simulink model "CorrectionAlgorithmHorizontalAndVertical"  (R2023a)
settings: Solver=FixedStepDiscrete  StartTime=0.0  StopTime=2  RelTol=1e-3
undefined symbols (not defined in the file or in its folder): gray
libraries: simulink x20, hdlsllib x10, visionsources x8, visionhdlio x6, dspsigops x4, visionhdlutilities x1
Description:
  | Sobel Edge Detection Using the MATLAB(R) Function Block
  | This example shows how to use HDL Coder(TM) to check,
  | generate, and verify HDL code for a Sobel Edge Detection
  | block built using the MATLAB Function block.
settings Model: Creator=The MathWorks, Inc.  LastModifiedBy=jms7664
settings SolverCC: AlgebraicLoopSolver=TrustRegion
settings DataIOCC: LimitDataPoints=on  SaveFormat=Array  SignalLogging=off  ReturnWorkspaceOutputs=off
settings OptimizationCC: BlockReduction=off  ConditionallyExecuteInputs=off  DefaultParameterBehavior=Inlined  ExpressionDepthLimit=2147483647  InitFltsAndDblsToZero=on  EfficientMapNaN2IntZero=off  LifeSpan=inf
settings DebuggingCC: AlgebraicLoopMsg=error  SaveWithParameterizedLinksMsg=none  UnderspecifiedInitializationDetection=Classic  MergeDetectMultiDrivingBlocksExec=none  SignalResolutionControl=TryResolveAllWithWarning  MultiTaskDSMMsg=warning  MultiTaskCondExecSysMsg=none  SingleTaskRateTransMsg=error  IntegerOverflowMsg=none  ParameterPrecisionLossMsg=none  FcnCallInpInsideContextMsg=warning  UnconnectedInputMsg=warning  UnconnectedOutputMsg=warning  UnconnectedLineMsg=warning  AllowSymbolicDim=off  StateNameClashWarn=warning  StrictBusMsg=ErrorOnBusTreatedAsVector  SFUnexpectedBacktrackingDiag=warning  SFNoUnconditionalDefaultTransitionDiag=warning  SFExecutionAtInitializationDiag=none  IntegerSaturationMsg=none  ArithmeticOperatorsInVariantConditions=warning
settings HardwareCC: ProdBitPerPointer=32  ProdBitPerSizeT=32  ProdBitPerPtrDiffT=32  ProdLargestAtomicFloat=None  ProdIntDivRoundTo=Undefined  ProdEndianess=Unspecified  ProdWordSize=32  ProdHWDeviceType=ASIC/FPGA  TargetHWDeviceType=32-bit Generic  ProdEqTarget=off
settings ModelReferenceCC: EnableRefExpFcnMdlSchedulingChecks=on  PropagateSignalLabelsOutOfModel=off
settings SFSimCC: SimUseLocalCustomCode=off  CustomCodeUndefinedFunction=UseInterfaceOnly
settings RTWCC: RTWUseLocalCustomCode=off  DLArmComputeVersion=19.05
settings CodeAppCC: StateflowObjectComments=on
settings GRTTargetCC: TargetFcnLib=ansi_tfl_tmw.mat  TargetLangStandard=C89/C90 (ANSI)  CombineOutputUpdateFcns=off  GRTInterface=on
settings ConfigComp: CovMetricSettings=dw  CovSaveCumulativeToWorkspaceVar=on  CovSaveSingleToWorkspaceVar=on  CovExternalEMLEnable=off

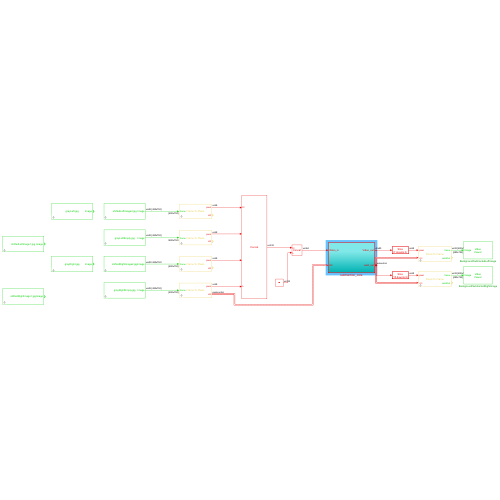
[thumbnail: Simulink's stored preview of the top-level diagram]
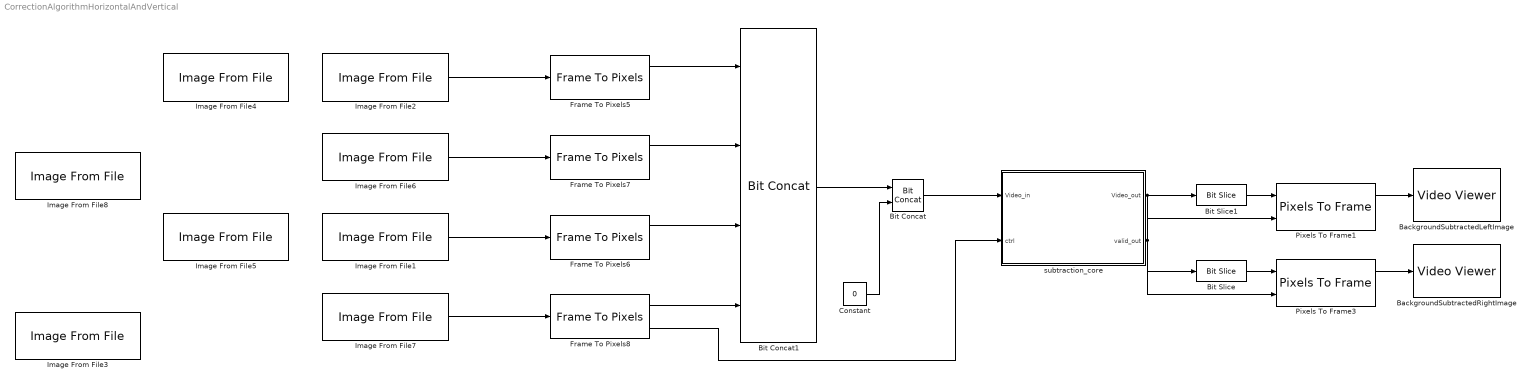
== system CorrectionAlgorithmHorizontalAndVertical ==
  BackgroundSubtractedLeftImage : VideoViewer  colormapValue=gray(256)  FigPos=[37 919 863 515]
  BackgroundSubtractedRightImage : VideoViewer  colormapValue=gray(256)  FigPos=[913 939 854 533]
  Bit Concat : hdlsllib/Logic and Bit Operations/Bit Concat  numInputs=2
  Bit Concat1 : hdlsllib/Logic and Bit Operations/Bit Concat  numInputs=4
  Bit Slice : hdlsllib/Logic and Bit Operations/Bit Slice  lidx=15  ridx=8
  Bit Slice1 : hdlsllib/Logic and Bit Operations/Bit Slice  lidx=7  ridx=0
  Constant : Constant  Value=0  OutDataTypeStr=uint32  SampleTime=-1
  Frame To Pixels{5..8} (4 alike) : visionhdlio/Frame To Pixels  NumComponents=1  NumPixels=1  VideoFormat=Custom  ActivePixelsPerLine=R  ActiveVideoLines=C  TotalPixelsPerLine=R  TotalVideoLines=C  StartingActiveLine=1  FrontPorch=0  SampleTime=0  VideoFormatCache=Custom  ActivePixelsPerLineCache=R  ActiveVideoLinesCache=C  TotalPixelsPerLineCache=R  TotalVideoLinesCache=C  StartingActiveLineCache=1  FrontPorchCache=0
  Image From File1 : visionsources/Image From File  Tag=vipblks_nd  FileName=shiftedRightImage2.jpg  Ts=1  imagePorts=One multidimensional signal  OutPortLabels=R|G|B  ImageDataType=Inherit from input image  sdImageDataType=uint(8)  Signed=on  WordLength=16  FractionLengthMode=User-defined  FractionLength=15
  Image From File2 : visionsources/Image From File  Tag=vipblks_nd  FileName=shiftedLeftImage2.jpg  Ts=1  imagePorts=One multidimensional signal  OutPortLabels=R|G|B  ImageDataType=Inherit from input image  sdImageDataType=uint(8)  Signed=on  WordLength=16  FractionLengthMode=User-defined  FractionLength=15
  Image From File3 : visionsources/Image From File  Tag=vipblks_nd  FileName=shiftedRightImage1.jpg  Ts=1  imagePorts=One multidimensional signal  OutPortLabels=R|G|B  ImageDataType=Inherit from input image  sdImageDataType=uint(8)  Signed=on  WordLength=16  FractionLengthMode=User-defined  FractionLength=15
  Image From File4 : visionsources/Image From File  Tag=vipblks_nd  FileName=grayLeft.jpg  Ts=1  imagePorts=One multidimensional signal  OutPortLabels=R|G|B  ImageDataType=Inherit from input image  sdImageDataType=uint(8)  Signed=on  WordLength=16  FractionLengthMode=User-defined  FractionLength=15
  Image From File5 : visionsources/Image From File  Tag=vipblks_nd  FileName=grayRight.jpg  Ts=1  imagePorts=One multidimensional signal  OutPortLabels=R|G|B  ImageDataType=Inherit from input image  sdImageDataType=uint(8)  Signed=on  WordLength=16  FractionLengthMode=User-defined  FractionLength=15
  Image From File6 : visionsources/Image From File  Tag=vipblks_nd  FileName=grayLeftEmpty.jpg  Ts=1  imagePorts=One multidimensional signal  OutPortLabels=R|G|B  ImageDataType=Inherit from input image  sdImageDataType=uint(8)  Signed=on  WordLength=16  FractionLengthMode=User-defined  FractionLength=15
  Image From File7 : visionsources/Image From File  Tag=vipblks_nd  FileName=grayRightEmpty.jpg  Ts=1  imagePorts=One multidimensional signal  OutPortLabels=R|G|B  ImageDataType=Inherit from input image  sdImageDataType=uint(8)  Signed=on  WordLength=16  FractionLengthMode=User-defined  FractionLength=15
  Image From File8 : visionsources/Image From File  Tag=vipblks_nd  FileName=shiftedLeftImage1.jpg  Ts=1  imagePorts=One multidimensional signal  OutPortLabels=R|G|B  ImageDataType=Inherit from input image  sdImageDataType=uint(8)  Signed=on  WordLength=16  FractionLengthMode=User-defined  FractionLength=15
  Pixels To Frame1 : visionhdlio/Pixels To Frame  NumComponents=1  NumPixels=1  VideoFormat=Custom  ActivePixelsPerLine=R  ActiveVideoLines=C  TotalPixelsPerLine=R  TotalVideoLines=C  VideoFormatCache=Custom  ActivePixelsPerLineCache=R  ActiveVideoLinesCache=C  TotalPixelsPerLineCache=R  TotalVideoLinesCache=C
  Pixels To Frame3 : visionhdlio/Pixels To Frame  NumComponents=1  NumPixels=1  VideoFormat=Custom  ActivePixelsPerLine=R  ActiveVideoLines=C  TotalPixelsPerLine=R  TotalVideoLines=C  VideoFormatCache=Custom  ActivePixelsPerLineCache=R  ActiveVideoLinesCache=C  TotalPixelsPerLineCache=R  TotalVideoLinesCache=C
  subtraction_core : Subsystem  TreatAsAtomicUnit=on
  wires:
  Image From File2/1 -> Frame To Pixels5/1
  Image From File6/1 -> Frame To Pixels7/1
  Image From File7/1 -> Frame To Pixels8/1
  Image From File1/1 -> Frame To Pixels6/1
  Frame To Pixels7/1 -> Bit Concat1/2
  Frame To Pixels5/1 -> Bit Concat1/1
  Frame To Pixels6/1 -> Bit Concat1/3
  Frame To Pixels8/1 -> Bit Concat1/4
  Frame To Pixels8/2 -> subtraction_core/2(ctrl)
  Bit Concat1/1 -> Bit Concat/1
  Constant/1 -> Bit Concat/2
  Bit Concat/1 -> subtraction_core/1(Video_in)
  subtraction_core/2(valid_out) -> Pixels To Frame3/2, Pixels To Frame1/2
  subtraction_core/1(Video_out) -> Bit Slice1/1, Bit Slice/1
  Bit Slice1/1 -> Pixels To Frame1/1
  Bit Slice/1 -> Pixels To Frame3/1
  Pixels To Frame1/1 -> BackgroundSubtractedLeftImage/1
  Pixels To Frame3/1 -> BackgroundSubtractedRightImage/1

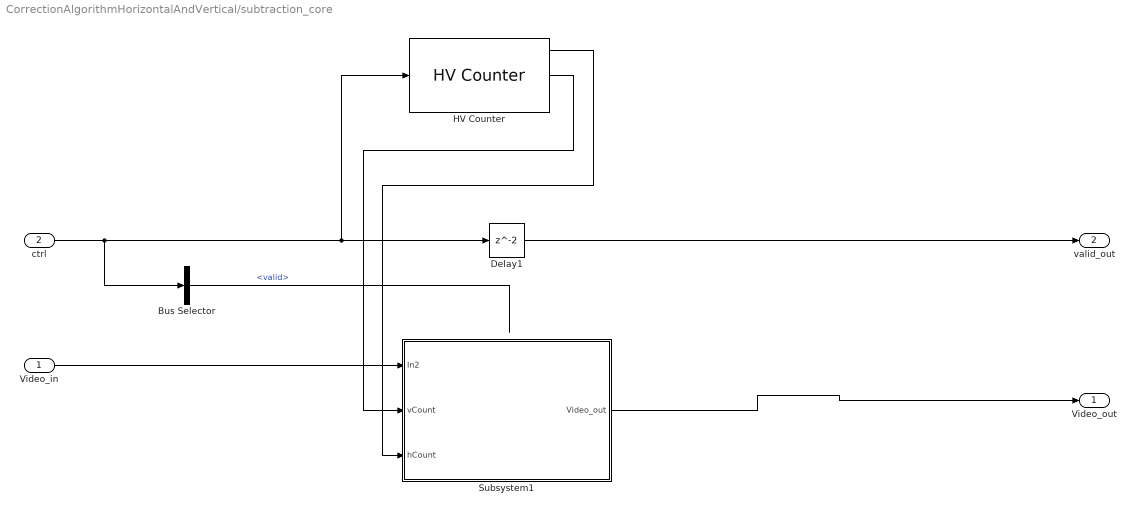
== system CorrectionAlgorithmHorizontalAndVertical/subtraction_core ==
  Video_in : Inport
  ctrl : Inport  Port=2
  Bus Selector : BusSelector  OutputSignals=valid
  Delay1 : Delay  InitialCondition=0
  HV Counter : visionhdlutilities/HV Counter  ActivePixelsPerLine=752  ActiveVideoLines=480  SimulateUsing=Code generation
  Subsystem1 : Subsystem
  Video_out : Outport  VectorParamsAs1DForOutWhenUnconnected=off
  valid_out : Outport  Port=2  VectorParamsAs1DForOutWhenUnconnected=off
  wires:
  Video_in/1 -> Subsystem1/1(In2)
  ctrl/1 -> Bus Selector/1, HV Counter/1, Delay1/1
  Bus Selector/1 -> ?  "<valid>"
  Subsystem1/1(Video_out) -> Video_out/1
  Delay1/1 -> valid_out/1
  HV Counter/1 -> Subsystem1/3(hCount)
  HV Counter/2 -> Subsystem1/2(vCount)

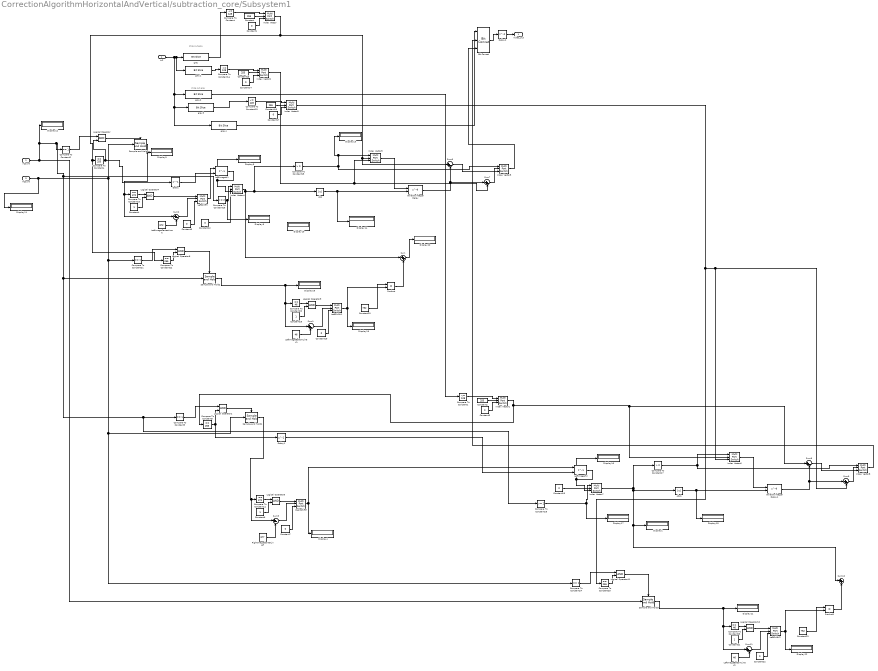
== system CorrectionAlgorithmHorizontalAndVertical/subtraction_core/Subsystem1 ==
  note: slice out gray
  note: slice out gray
  In2 : Inport
  vCount : Inport  Port=2
  hCount : Inport  Port=3
  Abs : Abs  SaturateOnIntegerOverflow=off
  Abs1 : Abs  SaturateOnIntegerOverflow=off
  Bit Concat : hdlsllib/Logic and Bit Operations/Bit Concat  numInputs=3
  Compare To Constant{,1,14,19} (4 alike) : simulink/Logic and Bit Operations/Compare To Constant  relop=<=  const=128  OutDataTypeStr=boolean
  Compare To Constant10 : simulink/Logic and Bit Operations/Compare To Constant  relop===  const=372  OutDataTypeStr=boolean
  Compare To Constant11 : simulink/Logic and Bit Operations/Compare To Constant  relop===  const=372  OutDataTypeStr=boolean
  Compare To Constant15 : simulink/Logic and Bit Operations/Compare To Constant  relop=>  const=0  OutDataTypeStr=boolean
  Compare To Constant16 : simulink/Logic and Bit Operations/Compare To Constant  relop=>=  const=2  OutDataTypeStr=boolean
  Compare To Constant17 : simulink/Logic and Bit Operations/Compare To Constant  relop=>  const=0  OutDataTypeStr=boolean
  Compare To Constant18 : simulink/Logic and Bit Operations/Compare To Constant  relop=>=  const=2  OutDataTypeStr=boolean
  Compare To Constant{2..3,21,24} (4 alike) : simulink/Logic and Bit Operations/Compare To Constant  relop===  const=1  OutDataTypeStr=boolean
  Compare To Constant20 : simulink/Logic and Bit Operations/Compare To Constant  relop===  const=46  OutDataTypeStr=boolean
  Compare To Constant{4..5,22,25} (4 alike) : simulink/Logic and Bit Operations/Compare To Constant  relop===  const=255  OutDataTypeStr=boolean
  Compare To Constant23 : simulink/Logic and Bit Operations/Compare To Constant  relop===  const=46  OutDataTypeStr=boolean
  Constant{,2,13,16} (4 alike) : Constant  Value=255  OutDataTypeStr=uint8
  Constant{1,3,5,7,12,14..15,17,19,22} (10 alike) : Constant  Value=0  OutDataTypeStr=int8
  Constant{4,6,18,21} (4 alike) : Constant
  Constant20 : Constant  Value=752
  Constant23 : Constant  Value=752
  Delay : Delay  DelayLength=1  InitialCondition=0
  Delay1 : Delay  DelayLength=1  InitialCondition=0
  Delay2 : Delay  InitialCondition=0
  Display{1,4..5,8..22} (18 alike) : Display
  Index Vector{,1..9} (10 alike) : MultiPortSwitch  DataPortOrder=Zero-based contiguous  Inputs=2  zeroidx=on  SaturateOnIntegerOverflow=off  InputSameDT=off
  LeftImageBottomLineV1 : Constant  Value=46
  LeftImageBottomLineV2 : Constant  Value=46
  LeftImageCenterLineH : Constant  Value=372
  LeftImageH1 : Delay  DelayLength=1  ShowEnablePort=on
      settings: InputPortMap=u0,e6
  LeftImageH2 : Delay  DelayLength=1  ShowEnablePort=on
      settings: InputPortMap=u0,e6
  LeftShiftH : MultiPortSwitch  DataPortOrder=Zero-based contiguous  Inputs=2  zeroidx=on  SaturateOnIntegerOverflow=off  InputSameDT=off
  LeftShiftV1 : MultiPortSwitch  DataPortOrder=Zero-based contiguous  Inputs=2  zeroidx=on  SaturateOnIntegerOverflow=off  InputSameDT=off
  LeftShiftV2 : MultiPortSwitch  DataPortOrder=Zero-based contiguous  Inputs=2  zeroidx=on  SaturateOnIntegerOverflow=off  InputSameDT=off
  Logical Operator{,1,4..5,8..11} (8 alike) : Logic  AllPortsSameDT=off  OutDataTypeStr=boolean
  Product : Product
  Product1 : Product
  RightImageCenterLineH : Constant  Value=377
  RightShiftH : MultiPortSwitch  DataPortOrder=Zero-based contiguous  Inputs=2  zeroidx=on  SaturateOnIntegerOverflow=off  InputSameDT=off
  Sample and Hold{,1..3} (4 alike) : dspsigops/Sample and Hold  trig=Falling edge  initCond=0  latchinput=on
  Sum : Sum  Inputs=|++
  Sum{1..3,11} (4 alike) : Sum  Inputs=|+-  OutDataTypeStr=int8  SaturateOnIntegerOverflow=on
  Sum10 : Sum  Inputs=|++
  Sum{6..9} (4 alike) : Sum  Inputs=|+-  OutDataTypeStr=uint8  SaturateOnIntegerOverflow=on
  Variable Integer Delay : Delay  DelayLengthSource=Input port
      settings: InputPortMap=u0,p1
  Variable Integer Delay1 : Delay  DelayLengthSource=Input port
      settings: InputPortMap=u0,p1
  gray : hdlsllib/Logic and Bit Operations/Bit Slice  lidx=63  ridx=56
  gray1 : hdlsllib/Logic and Bit Operations/Bit Slice  lidx=55  ridx=48
  gray2 : hdlsllib/Logic and Bit Operations/Bit Slice  lidx=47  ridx=40
  gray3 : hdlsllib/Logic and Bit Operations/Bit Slice  lidx=39  ridx=32
  gray4 : hdlsllib/Logic and Bit Operations/Bit Slice  lidx=63  ridx=32
  Video_out : Outport  InitialOutput=[0]
  wires:
  Bit Concat/1 -> Delay2/1
  Delay2/1 -> Video_out/1
  In2/1 -> gray4/1, gray3/1, gray2/1, gray1/1, gray/1
  Compare To Constant/1 -> Index Vector/1
  Constant/1 -> Index Vector/2
  Constant1/1 -> Index Vector/3
  Compare To Constant4/1 -> Logical Operator/2, Delay/1
  Compare To Constant5/1 -> Delay1/1, Logical Operator1/2
  Logical Operator1/1 -> Sample and Hold1/Trigger
  Compare To Constant3/1 -> Logical Operator1/1
  Constant3/1 -> Index Vector1/3
  Constant2/1 -> Index Vector1/2
  Compare To Constant1/1 -> Index Vector1/1
  gray2/1 -> Compare To Constant1/1
  gray/1 -> Compare To Constant/1
  Compare To Constant10/1 -> Logical Operator4/1
  Constant4/1 -> Logical Operator4/2
  Logical Operator4/1 -> LeftShiftH/1
  LeftImageCenterLineH/1 -> Sum2/2
  Sum2/1 -> LeftShiftH/2
  Constant5/1 -> LeftShiftH/3
  Constant7/1 -> RightShiftH/3
  Logical Operator5/1 -> RightShiftH/1
  Constant6/1 -> Logical Operator5/2
  Compare To Constant11/1 -> Logical Operator5/1
  Sum3/1 -> RightShiftH/2
  LeftShiftH/1 -> LeftImageH1/1
  RightImageCenterLineH/1 -> Sum3/2
  Compare To Constant14/1 -> Index Vector2/1
  Constant13/1 -> Index Vector2/2
  Constant14/1 -> Index Vector2/3
  gray1/1 -> Compare To Constant14/1
  Index Vector2/1 -> Sum7/2, Index Vector3/3
  Compare To Constant16/1 -> Display8/1, Index Vector4/1
  Constant12/1 -> Index Vector4/2
  Index Vector/1 -> Compare To Constant4/1, Compare To Constant22/1, Sum6/1, Index Vector3/2
  Compare To Constant15/1 -> Index Vector3/1, Display13/1, Index Vector5/1
  Sample and Hold/1 -> Sum2/1, Compare To Constant10/1, Display9/1
  Delay/1 -> LeftImageH1/2
  Compare To Constant2/1 -> Logical Operator/1
  Logical Operator/1 -> Sample and Hold/Trigger
  Index Vector3/1 -> Variable Integer Delay/1
  LeftImageH1/1 -> Index Vector4/3, Display5/1
  Abs/1 -> Display14/1, Variable Integer Delay/2
  Variable Integer Delay/1 -> Sum7/1, Sum6/2
  Sum6/1 -> Index Vector5/3
  Sum7/1 -> Index Vector5/2
  Sample and Hold1/1 -> Sum3/1, Compare To Constant11/1
  Sum8/1 -> Index Vector8/3
  Sum9/1 -> Index Vector8/2
  Variable Integer Delay1/1 -> Sum9/1, Sum8/2
  Compare To Constant17/1 -> Index Vector6/1, Index Vector8/1
  Constant15/1 -> Index Vector7/2
  Index Vector7/1 -> Sum10/1, Display1/1, Abs1/1, Compare To Constant17/1
  Compare To Constant18/1 -> Index Vector7/1, Display17/1
  RightShiftH/1 -> Display4/1, LeftImageH2/1
  Index Vector6/1 -> Variable Integer Delay1/1
  Abs1/1 -> Display15/1, Variable Integer Delay1/2
  LeftImageH2/1 -> Index Vector7/3, Display16/1
  Delay1/1 -> LeftImageH2/2
  Compare To Constant19/1 -> Index Vector9/1
  Constant17/1 -> Index Vector9/3
  Constant16/1 -> Index Vector9/2
  gray3/1 -> Compare To Constant19/1
  Compare To Constant21/1 -> Logical Operator8/1
  LeftImageBottomLineV1/1 -> Sum1/2
  Compare To Constant20/1 -> Logical Operator9/1
  LeftShiftV1/1 -> Display19/1, Product/2
  Compare To Constant22/1 -> Logical Operator8/2
  Constant19/1 -> LeftShiftV1/3
  Sum1/1 -> LeftShiftV1/2
  Constant18/1 -> Logical Operator9/2
  Logical Operator9/1 -> LeftShiftV1/1
  Sample and Hold2/1 -> Sum1/1, Compare To Constant20/1, Display18/1
  Logical Operator8/1 -> Sample and Hold2/Trigger
  Constant20/1 -> Product/1
  Product/1 -> Sum/2
  Sum/1 -> Display20/1
  Index Vector1/1 -> Sum8/1, Index Vector6/2, Compare To Constant5/1
  Index Vector4/1 -> Sum/1, Compare To Constant15/1, Abs/1
  Index Vector9/1 -> Compare To Constant25/1, Index Vector6/3, Sum9/2
  vCount/1 -> Sample and Hold3/1, Display12/1, Sample and Hold2/1, Compare To Constant18/1, Compare To Constant3/1, Compare To Constant16/1, Compare To Constant2/1
  Sample and Hold3/1 -> Sum11/1, Compare To Constant23/1, Display21/1
  Constant22/1 -> LeftShiftV2/3
  Product1/1 -> Sum10/2
  Constant23/1 -> Product1/1
  Constant21/1 -> Logical Operator10/2
  Compare To Constant24/1 -> Logical Operator11/1
  hCount/1 -> Sample and Hold/1, Compare To Constant21/1, Compare To Constant24/1, Sample and Hold1/1, Display11/1
  Logical Operator11/1 -> Sample and Hold3/Trigger
  Logical Operator10/1 -> LeftShiftV2/1
  Sum11/1 -> LeftShiftV2/2
  LeftImageBottomLineV2/1 -> Sum11/2
  LeftShiftV2/1 -> Display22/1, Product1/2
  Compare To Constant25/1 -> Logical Operator11/2
  Compare To Constant23/1 -> Logical Operator10/1
  gray4/1 -> Bit Concat/1
  Index Vector8/1 -> Bit Concat/2
  Index Vector5/1 -> Bit Concat/3
